simulink model "fuzzy_MATLAB_2012b"  (Simulink 8.0)
settings: Solver=ode3  StartTime=0.0  StopTime=500  FixedStep=0.1  RelTol=1e-3
libraries: fuzblock x1
settings Model: Creator=我爱计算宅  ModifiedByFormat=我爱计算宅  LastModifiedBy=我爱计算宅  ModifiedComment=我爱计算宅 -- 我爱计算宅 -- Version 1.37
settings Model: ModifiedHistory=|
  | 我爱计算宅 -- 我爱计算宅 -- Version 1.37
  | 
  | 我爱计算宅 -- 我爱计算宅 -- Version 1.37
settings SolverCC: ZeroCrossControl=DisableAll
settings DataIOCC: SignalLoggingSaveFormat=ModelDataLogs
settings OptimizationCC: ExpressionDepthLimit=128  InitFltsAndDblsToZero=on
settings DebuggingCC: SaveWithParameterizedLinksMsg=none  SignalResolutionControl=TryResolveAllWithWarning  MultiTaskDSMMsg=warning  MultiTaskCondExecSysMsg=none  FcnCallInpInsideContextMsg=EnableAllAsWarning  FrameProcessingCompatibilityMsg=error  StateNameClashWarn=none
settings CodeAppCC: CustomSymbolStrType=$N$R$M_T
settings GRTTargetCC: TargetFcnLib=ansi_tfl_tmw.mat  CodeReplacementLibrary=C89/C90 (ANSI)  GeneratePreprocessorConditionals=Use local settings  CombineOutputUpdateFcns=off  GRTInterface=on

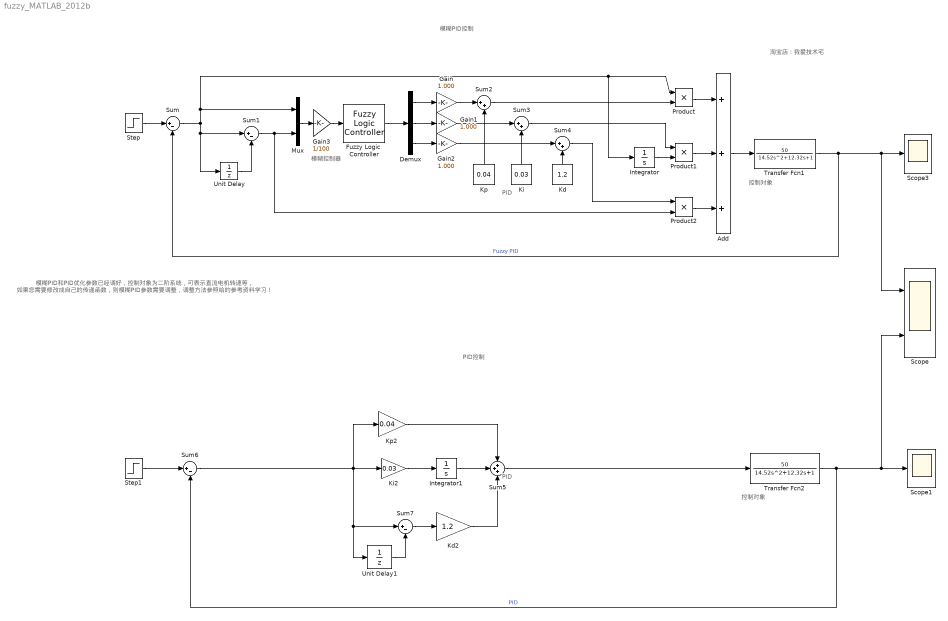
== system fuzzy_MATLAB_2012b ==
  note: 模糊PID和PID优化参数已经调好，控制对象为二阶系统，可表示直流电机转速等，
      | 如果您需要修改成自己的传递函数，则模糊PID参数需要调整，调整方法参照给的参考资料学习！
  note: 淘宝店：我爱技术宅
  note: 模糊PID控制
  note: PID控制
  note: 控制对象
  note: 控制对象
  note: 模糊控制器
  note: PID
  note: PID
  Add : Sum  Inputs=3
  Demux : Demux  Outputs=3
  Fuzzy Logic  Controller : fuzblock/Fuzzy Logic  Controller  FIS='fuzzypid.fis'
  Gain : Gain  Gain=1.000
  Gain1 : Gain  Gain=1.000
  Gain2 : Gain  Gain=1.000
  Gain3 : Gain  Gain=1/100
  Integrator : Integrator
  Integrator1 : Integrator
  Kd : Constant  Value=1.2
  Kd2 : Gain  Gain=1.2
  Ki : Constant  Value=0.03
  Ki2 : Gain  Gain=0.03
  Kp : Constant  Value=0.04
  Kp2 : Gain  Gain=0.04
  Mux : Mux  Inputs=2
  Product : Product
  Product1 : Product
  Product2 : Product
  Scope : Scope  NumInputPorts=2
      settings: TimeRange=auto  ShowLegends=on  MaxDataPoints=5000  SaveToWorkspace=off  SaveName=ScopeData  YMin=-17.69091~-5  YMax=159.21819~5  SampleTime=-1
  Scope1 : Scope
      settings: TimeRange=auto  ShowLegends=on  MaxDataPoints=5000  SaveToWorkspace=off  YMin=-17.69091  YMax=159.21819  SampleTime=-1
  Scope3 : Scope
      settings: TimeRange=auto  ShowLegends=on  MaxDataPoints=5000  SaveToWorkspace=off  SaveName=ScopeData3  YMin=-13.37167  YMax=120.34507  SampleTime=-1
  Step : Step  Time=0  After=100  SampleTime=0
  Step1 : Step  Time=0  After=100  SampleTime=0
  Sum{,1,6..7} (4 alike) : Sum  Inputs=|+-
  Sum2 : Sum  Inputs=|++
  Sum3 : Sum  Inputs=|++
  Sum4 : Sum  Inputs=|++
  Sum5 : Sum  Inputs=+++
  Transfer Fcn1 : TransferFcn  Numerator=[50]  Denominator=[14.52 12.32 1]
  Transfer Fcn2 : TransferFcn  Numerator=[50]  Denominator=[14.52 12.32 1]
  Unit Delay : UnitDelay  SampleTime=-1  HasFrameUpgradeWarning=on
  Unit Delay1 : UnitDelay  SampleTime=-1  HasFrameUpgradeWarning=on
  wires:
  Step/1 -> Sum/1
  Sum/1 -> Unit Delay/1, Sum1/1, Integrator/1, Product/1, Mux/1
  Mux/1 -> Gain3/1
  Unit Delay/1 -> Sum1/2
  Sum1/1 -> Product2/2, Mux/2
  Fuzzy Logic  Controller/1 -> Demux/1
  Demux/1 -> Gain/1
  Kp/1 -> Sum2/2
  Demux/2 -> Gain1/1
  Ki/1 -> Sum3/2
  Kd/1 -> Sum4/2
  Sum2/1 -> Product/2
  Sum3/1 -> Product1/1
  Integrator/1 -> Product1/2
  Transfer Fcn1/1 -> Scope3/1, Scope/1, Sum/2  "Fuzzy PID"
  Sum4/1 -> Product2/1
  Product2/1 -> Add/3
  Product1/1 -> Add/2
  Product/1 -> Add/1
  Add/1 -> Transfer Fcn1/1
  Ki2/1 -> Integrator1/1
  Integrator1/1 -> Sum5/2
  Kp2/1 -> Sum5/1
  Sum5/1 -> Transfer Fcn2/1
  Unit Delay1/1 -> Sum7/2
  Sum6/1 -> Unit Delay1/1, Sum7/1, Kp2/1, Ki2/1
  Sum7/1 -> Kd2/1
  Step1/1 -> Sum6/1
  Transfer Fcn2/1 -> Sum6/2, Scope1/1, Scope/2  "PID"
  Kd2/1 -> Sum5/3
  Demux/3 -> Gain2/1
  Gain1/1 -> Sum3/1
  Gain/1 -> Sum2/1
  Gain2/1 -> Sum4/1
  Gain3/1 -> Fuzzy Logic  Controller/1
